simulink model "keyboardDriver"  (R2024a)
settings: Solver=FixedStepDiscrete  StartTime=0.0  StopTime=inf  FixedStep=1/500  RelTol=1e-3  EnableMultiTasking=on
undefined symbols (not defined in the file or in its folder): Host
libraries: quarc_library x5, simulink x2
settings Model: ExtModeTrigDuration=10000  Creator=mbohra  LastModifiedBy=mbohra
settings SolverCC: AlgebraicLoopSolver=TrustRegion  PositivePriorityOrder=on
settings DataIOCC: ReturnWorkspaceOutputs=off
settings DebuggingCC: UnconnectedInputMsg=warning  UnconnectedOutputMsg=warning  UnconnectedLineMsg=warning  ArithmeticOperatorsInVariantConditions=warning
settings ModelReferenceCC: EnableRefExpFcnMdlSchedulingChecks=on
settings SFSimCC: SimUseLocalCustomCode=off  CustomCodeUndefinedFunction=UseInterfaceOnly
settings RTWCC: Description=QUARC Win64 Target Using Toolchain  SystemTargetFile=quarc_win64.tlc  TemplateMakefile=quarc_default_tmf  RTWUseLocalCustomCode=off  Toolchain=QUARC win64 | nmake (64-bit Windows)  BuildConfiguration=Faster Runs  GPUComputeCapability=3.5
settings CodeAppCC: StateflowObjectComments=on
settings STFCustomTargetCC: ConcurrentExecutionCompliant=on  SystemTargetFile=quarc_win64.tlc
settings GRTTargetCC: ParMdlRefBuildCompliant=off  CompOptLevelCompliant=off  CombineOutputUpdateFcns=off  MatFileLogging=off  CPPClassGenCompliant=off  GRTInterface=on  ExtMode=on  ExtModeMexFile=quarc_comm
settings ConfigComp: CovMetricSettings=dswe

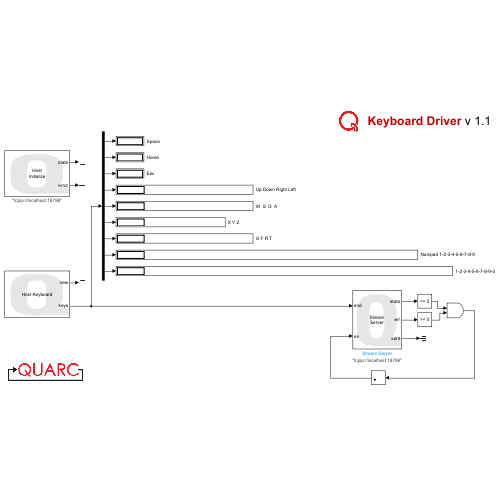
[thumbnail: Simulink's stored preview of the top-level diagram]
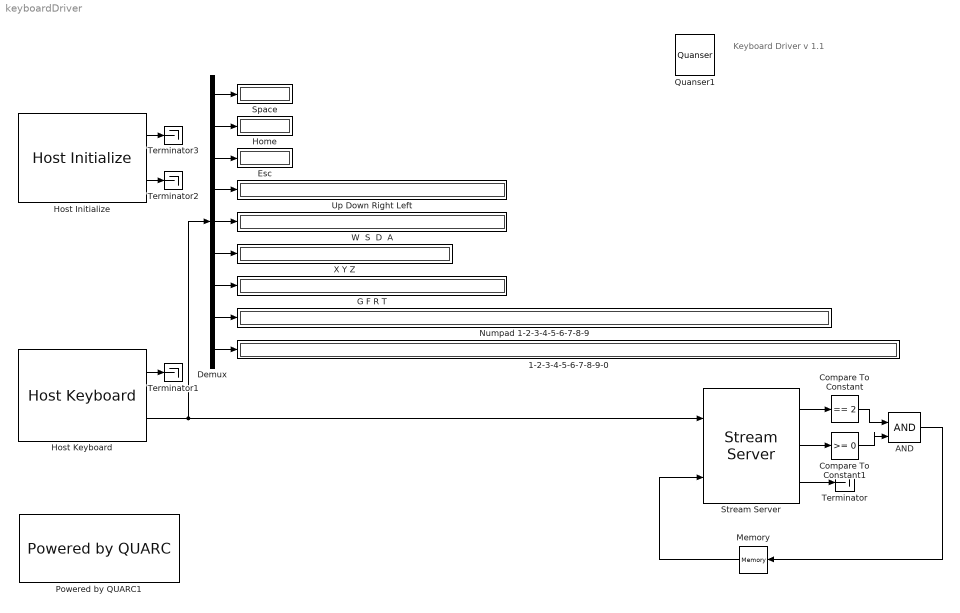
== system keyboardDriver ==
  note: Keyboard Driver v 1.1
  1-2-3-4-5-6-7-8-9-0 : Display
  AND : Logic  IconShape=distinctive  AllPortsSameDT=off  OutDataTypeStr=boolean
  Compare To Constant : simulink/Logic and Bit Operations/Compare To Constant  relop===  const=2  OutDataTypeStr=boolean
  Compare To Constant1 : simulink/Logic and Bit Operations/Compare To Constant  relop=>=  const=0  OutDataTypeStr=boolean
  Demux : Demux  Outputs=[1 1 1 4 4 3 4 9 10]
  Esc : Display
  G F R T : Display
  Home : Display
  Host Initialize : quarc_library/Devices/Peripherals/Host/Host Initialize  object_name=Host-1  uri_source=Specify via dialog (do not evaluate)  uri=tcpip://localhost:18798  send_buffer_size=1000  receive_buffer_size=1000  thread_priority=0  run_client=on  use_window=off  window_position=[]  sample_time=qc_get_step_size  active=on
      settings: AttributesFormatString="\"tcpip://localhost:18798\""  SourceProductName=QUARC Targets
  Host Keyboard : quarc_library/Devices/Peripherals/Host/Host Keyboard  object_name=Host-1  virtual_key="[32   36   27   38   40   39   37   87   83   68   65   88   89   90   71   70   82   84   97   98   99  100  101  102  103  104  105   49   50   51   52   53   54   55   56   57   48]"  sample_time=qc_get_step_size  enabled=on  debug_mode=off
      settings: SourceProductName=QUARC Targets
  Memory : Memory
  "Numpad 1-2-3-4-5-6-7-8-9 " : Display
  Powered by QUARC1 : quarc_library/Logos/Powered by QUARC
  Quanser1 : quarc_library/Logos/Quanser
  Space : Display
  Stream Server : quarc_library/Communications/Basic/Stream Server  uri_source=Specify via dialog (do not evaluate)  uri=tcpip://localhost:18799  send_buffer_size=1460  receive_buffer_size=1460  byte_order=little endian (Intel - LSB first)  optimization=Minimum latency  send_options=Send most recent data  receive_options=Do not receive data  default_value=[0]  sample_time=qc_get_step_size  active=on  implementation=Use blocking I/O in a separate thread  send_fifo_size=1000  receive_fifo_size=1000  send_priority=0  receive_priority=0  send_dimensions=off  receive_dimensions=off  max_dimensions=-1  data_type=Inherited via back propagation  type_expr=BusObject
      settings: AttributesFormatString="\"tcpip://localhost:18799\""
  Terminator{,1..3} (4 alike) : Terminator
  Up Down Right Left : Display
  W  S  D  A : Display
  X Y Z : Display
  wires:
  Host Keyboard/2 -> Demux/1, Stream Server/1
  Stream Server/1 -> Compare To Constant/1
  Stream Server/2 -> Compare To Constant1/1
  Compare To Constant/1 -> AND/1
  Compare To Constant1/1 -> AND/2
  AND/1 -> Memory/1
  Memory/1 -> Stream Server/2
  Stream Server/3 -> Terminator/1
  Demux/7 -> G F R T/1
  Demux/1 -> Space/1
  Demux/2 -> Home/1
  Demux/3 -> Esc/1
  Demux/4 -> Up Down Right Left/1
  Demux/5 -> W  S  D  A/1
  Demux/6 -> X Y Z/1
  Host Keyboard/1 -> Terminator1/1
  Host Initialize/2 -> Terminator2/1
  Host Initialize/1 -> Terminator3/1
  Demux/8 -> "Numpad 1-2-3-4-5-6-7-8-9 "/1
  Demux/9 -> 1-2-3-4-5-6-7-8-9-0/1
